simulink model "Model_1a_H2_clean"  (R2019a)
settings: Solver=FixedStepAuto  StartTime=0.0  StopTime=8760  FixedStep=1  RelTol=1e-3
libraries: simulink x7
settings Model: Creator=senja  LastModifiedBy=senja

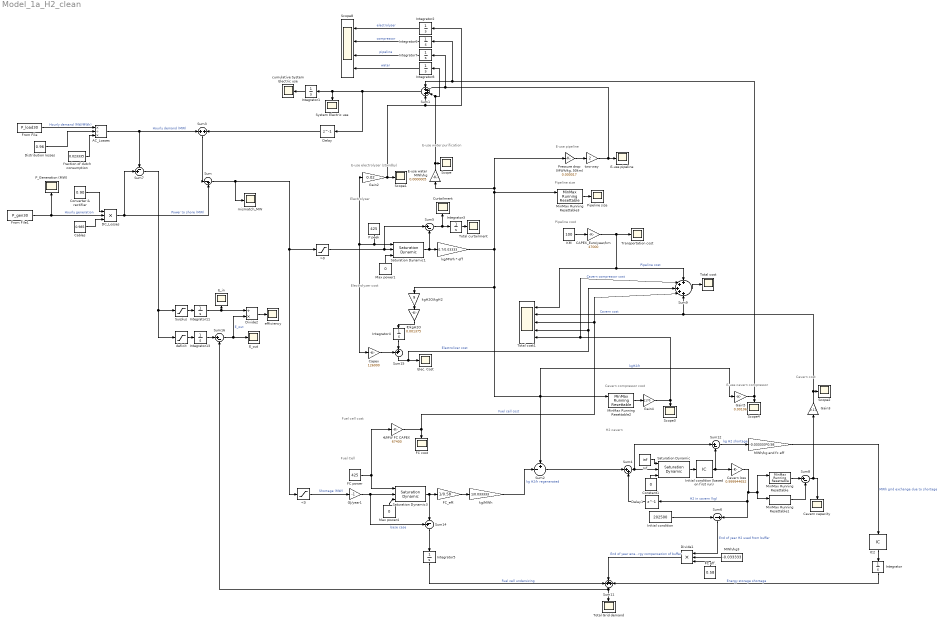
== system Model_1a_H2_clean ==
  note: Pipeline size
  note: E-use pipeline
  note: E-use cavern compressor
  note: Cavern compressor cost
  note: Cavern cost
  note: E-use electrolyser (standby)
  note: E-use water purification
  note: Fuel cell cost
  note: Pipeline cost
  note: H2 cavern
  note: Fuel Cell
  note: Electrolyser
  note: Electrolyzer cost
  <0 : Saturate  UpperLimit=0  LowerLimit=-inf
  >0 : Saturate  UpperLimit=inf  LowerLimit=0
  AC_Losses : Product  Inputs=*/*
  CAPEX_Euro/year/km : Gain  Gain=47000
  Cables : Constant  Value=0.985
  Capex : Gain  Gain=126000
  Cavern capacity : Scope
  Cavern loss : Gain  Gain=0.999944652
  Constant1 : Constant  Value=0
  Converter & rectifier : Constant  Value=0.90
  Curtailment : Scope
  DC_Losses : Product  Inputs=3
  Delay : Delay  DelayLength=1  InitialCondition=0
  Delay1 : Delay  DelayLength=1  InitialCondition=0
  Distribution losses : Constant  Value=0.96
  Divide1 : Product  Inputs=***
  Divide2 : Product  Inputs=/*
  E-use pipeline : Scope
  E-use water MWh/kg : Gain  Gain=0.0000005
  "E_in " : Scope
  E_out : Scope
  Elec. Cost : Scope
  FC cost : Scope
  FC eff. : Constant  Value=0.58
  FC power : Constant  Value=425
  FC_eff. : Gain  Gain=1/0.58
  From File : FromFile  FileName=P_load30  SampleTime=0
  From File1 : FromFile  FileName=P_gen30  SampleTime=0
  GJ/year1 : Gain  Gain=-1
  Gain2 : Gain  Gain=0.02
  Gain3 : Gain  Gain=0.17
  Gain4 : Gain  Gain=1170
  Gain5 : Gain  Gain=0.00106
  IC2 : InitialCondition  Value=0
  Inf : Constant  Value=inf  OutDataTypeStr=Inherit: Inherit via back propagation
  Initial condition : Constant  Value=202500
  Initial condition (based on first run) : InitialCondition  Value=202500
  Integrator{,1..8,11,13} (11 alike) : Integrator
  KM : Constant  Value=100
  MWh/kg and fc eff : Gain  Gain=-0.033333*0.58
  MWh/kg3 : Constant  Value=-0.033333
  Max power1 : Constant  Value=0
  Max power4 : Constant  Value=0
  MinMax Running Resettable : simulink/Math Operations/MinMax Running Resettable  Function=max  vinit=0.0
  MinMax Running Resettable1 : simulink/Math Operations/MinMax Running Resettable  Function=min  vinit=0.0
  MinMax Running Resettable2 : simulink/Math Operations/MinMax Running Resettable  Function=max  vinit=0.0
  MinMax Running Resettable3 : simulink/Math Operations/MinMax Running Resettable  Function=max  vinit=0.0
  P peek : Constant  Value=425
  P_Generation (MW) : Scope
  Pipeline size : Scope
  "Pressure drop (MWh/kg, 50km)" : Gain  Gain=0.000017
  Saturation Dynamic : simulink/Discontinuities/Saturation Dynamic  OutMin=0  OutMax=[]  OutDataTypeStr=Inherit: Same as second input  OutDataType=fixdt(1, 16)  OutScaling=2^-10  DoSatur=off
  Saturation Dynamic1 : simulink/Discontinuities/Saturation Dynamic  OutMin=[]  OutMax=[]  OutDataTypeStr=Inherit: Same as second input  OutDataType=fixdt(1, 16)  OutScaling=2^-10  DoSatur=off
  Saturation Dynamic3 : simulink/Discontinuities/Saturation Dynamic  OutMin=[]  OutMax=[]  OutDataTypeStr=Inherit: Same as second input  OutDataType=fixdt(1, 16)  OutScaling=2^-10  DoSatur=off
  Scope{,1..4} (5 alike) : Scope
  Scope8 : Scope  NumInputPorts=4
  Sum : Sum  Inputs=|-+
  Sum1 : Sum  Inputs=++++
  Sum11 : Sum  Inputs=+++
  Sum{5,8,12,16} (4 alike) : Sum  Inputs=|+-
  Sum14 : Sum  Inputs=+-|
  Sum15 : Sum  Inputs=++|
  Sum2 : Sum  Inputs=+-|
  Sum3 : Sum  Inputs=+|+
  Sum4 : Sum  Inputs=|++
  Sum6 : Sum  Inputs=-|+
  Sum7 : Sum  Inputs=-+|
  Sum9 : Sum  Inputs=+++++
  Surplus : Saturate  UpperLimit=inf  LowerLimit=0
  System Electric use : Scope
  Total Grid demand : Scope
  Total cost : Scope
  Total cost1 : Scope  NumInputPorts=5
  Total curtailment : Scope
  Transportation cost : Scope
  cumulative System Electric use : Scope
  deficit : Saturate  UpperLimit=inf  LowerLimit=0
  efficiency : Scope
  fraction of dutch consumption : Constant  Value=0.023335
  kg/MWh : Gain  Gain=1/0.033333
  kg/MWh * eff : Gain  Gain=0.7/0.03333
  kgH2O/kgH2 : Gain  Gain=9
  mismatch_MW : Scope
  two-way : Gain  Gain=2
  €/MW FC CAPEX : Gain  Gain=67400
  €/kgH2O : Gain  Gain=0.001375
  wires:
  From File/1 -> AC_Losses/1  "Hourly demand (MW/MWh)"
  fraction of dutch consumption/1 -> AC_Losses/3
  Distribution losses/1 -> AC_Losses/2
  Cables/1 -> DC_Losses/3
  Converter & rectifier/1 -> DC_Losses/1
  DC_Losses/1 -> Sum7/2, Sum/2  "Power to shore (MW)"
  <0/1 -> GJ/year1/1  "Shortage (MW)"
  AC_Losses/1 -> Sum3/1, Sum7/1  "Hourly demand (MW)"
  From File1/1 -> P_Generation (MW)/1, DC_Losses/2  "Hourly generation"
  Max power1/1 -> Saturation Dynamic1/3
  Capex/1 -> Sum15/1
  Sum15/1 -> Elec. Cost/1, Sum9/3, Total cost1/4  "Electrolizer cost"
  €/kgH2O/1 -> Integrator4/1
  P peek/1 -> Gain2/1, Capex/1, Saturation Dynamic1/1
  GJ/year1/1 -> Sum14/1, Saturation Dynamic3/2  "base case"
  KM/1 -> CAPEX_Euro/year/km/1
  CAPEX_Euro/year/km/1 -> Total cost1/1, Sum9/1, Transportation cost/1  "Pipeline cost"
  kg/MWh * eff/1 -> E-use water MWh/kg/1, "Pressure drop (MWh/kg, 50km)"/1, MinMax Running Resettable3/1, MinMax Running Resettable2/1, Sum2/1, Gain5/1, kgH2O/kgH2/1  "kgH2/h"
  Sum9/1 -> Total cost/1
  FC power/1 -> Saturation Dynamic3/1, €/MW FC CAPEX/1
  Max power4/1 -> Saturation Dynamic3/3
  Saturation Dynamic3/1 -> Sum14/2, FC_eff./1
  kg/MWh/1 -> Sum2/2  "kg H2/h regenerated"
  Integrator3/1 -> Total curtailment/1
  kgH2O/kgH2/1 -> €/kgH2O/1
  Integrator4/1 -> Sum15/2
  €/MW FC CAPEX/1 -> Sum9/4, Total cost1/3, FC cost/1  "Fuel cell cost"
  MinMax Running Resettable/1 -> Sum8/1
  MinMax Running Resettable1/1 -> Sum8/2
  Sum8/1 -> Cavern capacity/1, Gain3/1
  Sum5/1 -> Integrator3/1, Curtailment/1
  MWh/kg and fc eff/1 -> IC2/1  "MWh grid exchange due to shortage"
  Sum14/1 -> Integrator5/1
  Initial condition/1 -> Sum6/1
  Integrator5/1 -> Sum11/1  "Fuel cell undersizing"
  Sum6/1 -> Divide1/1  "End of year H2 used from buffer"
  E-use water MWh/kg/1 -> Integrator8/1, Sum1/3, Scope/1
  Gain2/1 -> Scope1/1, Integrator2/1, Sum1/4
  Gain3/1 -> Total cost1/2, Sum9/5, Scope2/1  "Cavern cost"
  MinMax Running Resettable2/1 -> Gain4/1
  Gain4/1 -> Scope3/1, Total cost1/5, Sum9/2  "Cavern compressor cost"
  Gain5/1 -> Sum1/1, Integrator6/1, Scope4/1
  "Pressure drop (MWh/kg, 50km)"/1 -> two-way/1
  two-way/1 -> Sum1/2, Integrator7/1, E-use pipeline/1
  Sum3/1 -> Sum/1
  Sum1/1 -> Delay/1, Integrator1/1, System Electric use/1
  Delay/1 -> Sum3/2
  Integrator1/1 -> cumulative System Electric use/1
  MWh/kg3/1 -> Divide1/2
  FC eff./1 -> Divide1/3
  Divide1/1 -> Sum11/2  "End of year energy compensation of buffer"
  Cavern loss/1 -> Sum6/2, Delay1/1, MinMax Running Resettable/1, MinMax Running Resettable1/1  "H2 in cavern (kg)"
  Integrator/1 -> Sum11/3  "Energy storage shortage"
  Sum12/1 -> MWh/kg and fc eff/1  "kg H2 shortage"
  Delay1/1 -> Sum4/2
  Constant1/1 -> Saturation Dynamic/3
  Saturation Dynamic/1 -> Initial condition (based on first run)/1
  Sum4/1 -> Sum12/1, Saturation Dynamic/2
  Initial condition (based on first run)/1 -> Cavern loss/1, Sum12/2
  Sum2/1 -> Sum4/1
  Inf/1 -> Saturation Dynamic/1
  IC2/1 -> Integrator/1
  Integrator2/1 -> Scope8/1  "electrolyser"
  Integrator6/1 -> Scope8/2  "compressor"
  Integrator7/1 -> Scope8/3  "pipeline"
  Integrator8/1 -> Scope8/4  "water"
  Sum7/1 -> deficit/1, Surplus/1
  Surplus/1 -> Integrator11/1
  deficit/1 -> Integrator13/1
  Integrator13/1 -> Sum16/1
  Sum16/1 -> Divide2/2, E_out/1  "E_out"
  Saturation Dynamic1/1 -> kg/MWh * eff/1, Sum5/2
  FC_eff./1 -> kg/MWh/1
  Integrator11/1 -> Divide2/1, "E_in "/1
  Divide2/1 -> efficiency/1
  Sum11/1 -> Total Grid demand/1, Sum16/2
  >0/1 -> Sum5/1, Saturation Dynamic1/2
  Sum/1 -> <0/1, >0/1, mismatch_MW/1
  MinMax Running Resettable3/1 -> Pipeline size/1
